simulink model "Sim"  (R2023a)
settings: Solver=FixedStepAuto  StartTime=0.0  StopTime=20  FixedStep=1e-4  RelTol=1e-3
values from neighbouring files (symbols this model uses):
  A1 = 28e-4    (= 0.0028)    [main.m]    (also in main2.m; main3.m; main4.m)
  a1 = 0.071e-4    (= 7.1e-06)    [main.m]    (also in main2.m; main3.m; main4.m)
  A2 = 32e-4    (= 0.0032)    [main.m]    (also in main2.m; main3.m; main4.m)
  a2 = 0.057e-4    (= 5.7e-06)    [main.m]    (also in main2.m; main3.m; main4.m)
  a3 = 0.071e-4    (= 7.1e-06)    [main.m]    (also in main2.m; main3.m; main4.m)
  A3 = 28e-4    (= 0.0028)    [main.m]    (also in main2.m; main3.m; main4.m)
  A4 = 32e-4    (= 0.0032)    [main.m]    (also in main2.m; main3.m; main4.m)
  a4 = 0.057e-4    (= 5.7e-06)    [main.m]    (also in main2.m; main3.m; main4.m)
  Com_V1 = 1.1*V01    (= 3.3)    [main.m]
  Com_V2 = 1.1*V02    (= 3.3)    [main.m]
  delay_Com_V1 = 2.5    [main.m]
  delay_Com_V2 = 1.5    [main.m]
  g = 9.81    [main.m]    (also in main2.m; main3.m; main4.m)
  gamma1 = 0.7    [main.m]    (also in main2.m; main3.m; main4.m)
  gamma2 = 0.6    [main.m]    (also in main2.m; main3.m; main4.m)
  H01 = (gamma1*k1*V01+(1-gamma2)*k2*V02)/(a1*sqrt(2*g))    [main.m]    (also in main2.m; main3.m; main4.m)
  H02 = (gamma2*k2*V02+(1-gamma1)*k1*V01)/(a2*sqrt(2*g))    [main.m]    (also in main2.m; main3.m; main4.m)
  H03 = (1-gamma2)*k2*V02/(a3*sqrt(2*g))    [main.m]    (also in main2.m; main3.m; main4.m)
  H04 = (1-gamma1)*k1*V01/(a4*sqrt(2*g))    [main.m]    (also in main2.m; main3.m; main4.m)
  k1 = 3.33e-6    (= 3.33e-06)    [main.m]    (also in main2.m; main3.m; main4.m)
  k2 = 3.35e-6    (= 3.35e-06)    [main.m]    (also in main2.m; main3.m; main4.m)
  Matrix_dX_U = [gamma1*k1/A1, 0 ... (first row only)    [main.m]    (also in main2.m; main3.m; main4.m)
  Matrix_dX_X = [-1/T1, 0, -A3/(A1*T3), 0 ... (first row only)    [main.m]    (also in main2.m; main3.m; main4.m)
  Matrix_H0 = [H01^2;H02^2;H03^2;H04^2]    [main.m]    (also in main2.m; main3.m; main4.m)
  Matrix_V0 = [V01;V02]    [main.m]    (also in main2.m; main3.m; main4.m)
  V01 = 3    [main.m]    (also in main2.m; main3.m; main4.m)
  V02 = 3    [main.m]    (also in main2.m; main3.m; main4.m)
settings Model: Creator=philippecasteres  LastModifiedBy=philippecasteres

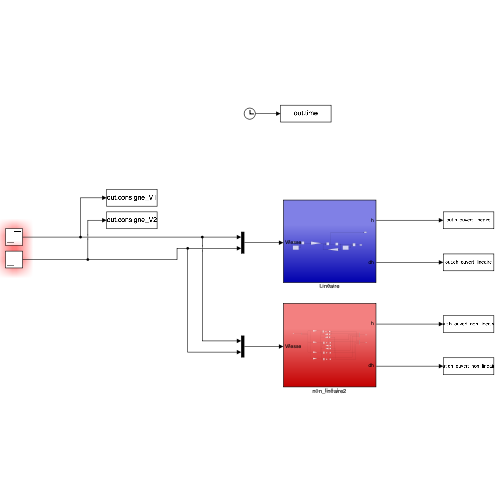
[thumbnail: Simulink's stored preview of the top-level diagram]
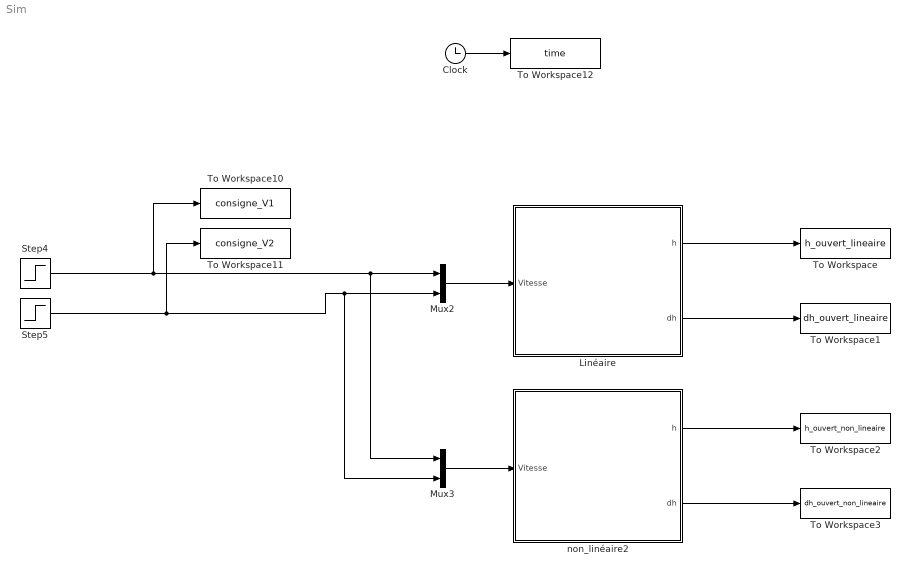
== system Sim ==
  Clock : Clock
  Linéaire : Subsystem
  Mux2 : Mux  Inputs=2
  Mux3 : Mux  Inputs=2
  Step4 : Step  Time=delay_Com_V1  Before=V01  After=Com_V1  SampleTime=0
  Step5 : Step  Time=delay_Com_V2  Before=V02  After=Com_V2  SampleTime=0
  To Workspace : ToWorkspace  VariableName=h_ouvert_lineaire  SaveFormat=Timeseries  SampleTime=-1
  To Workspace1 : ToWorkspace  VariableName=dh_ouvert_lineaire  SaveFormat=Timeseries  SampleTime=-1
  To Workspace10 : ToWorkspace  VariableName=consigne_V1  SaveFormat=Timeseries  SampleTime=-1
  To Workspace11 : ToWorkspace  VariableName=consigne_V2  SaveFormat=Timeseries  SampleTime=-1
  To Workspace12 : ToWorkspace  VariableName=time  SaveFormat=Timeseries  SampleTime=-1
  To Workspace2 : ToWorkspace  VariableName=h_ouvert_non_lineaire  SaveFormat=Timeseries  SampleTime=-1
  To Workspace3 : ToWorkspace  VariableName=dh_ouvert_non_lineaire  SaveFormat=Timeseries  SampleTime=-1
  non_linéaire2 : Subsystem
  wires:
  Step5/1 -> To Workspace11/1, Mux3/2, Mux2/2
  Step4/1 -> To Workspace10/1, Mux3/1, Mux2/1
  Linéaire/1(h) -> To Workspace/1
  Linéaire/2(dh) -> To Workspace1/1
  Mux2/1 -> Linéaire/1(Vitesse)
  non_linéaire2/2(dh) -> To Workspace3/1
  non_linéaire2/1(h) -> To Workspace2/1
  Mux3/1 -> non_linéaire2/1(Vitesse)
  Clock/1 -> To Workspace12/1

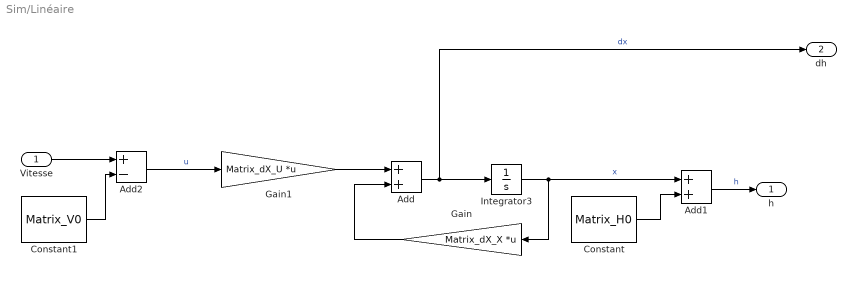
== system Sim/Linéaire ==
  Vitesse : Inport
  Add : Sum
  Add1 : Sum
  Add2 : Sum  Inputs=+-
  Constant : Constant  Value=Matrix_H0
  Constant1 : Constant  Value=Matrix_V0
  Gain : Gain  Gain=Matrix_dX_X  Multiplication=Matrix(K*u)
  Gain1 : Gain  Gain=Matrix_dX_U  Multiplication=Matrix(K*u) (u vector)
  Integrator3 : Integrator
  h : Outport
  dh : Outport  Port=2
  wires:
  Constant/1 -> Add1/2
  Add1/1 -> h/1  "h"
  Add2/1 -> Gain1/1  "u"
  Vitesse/1 -> Add2/1
  Gain/1 -> Add/2
  Constant1/1 -> Add2/2
  Gain1/1 -> Add/1
  Add/1 -> Integrator3/1, dh/1  "dx"
  Integrator3/1 -> Add1/1, Gain/1  "x"

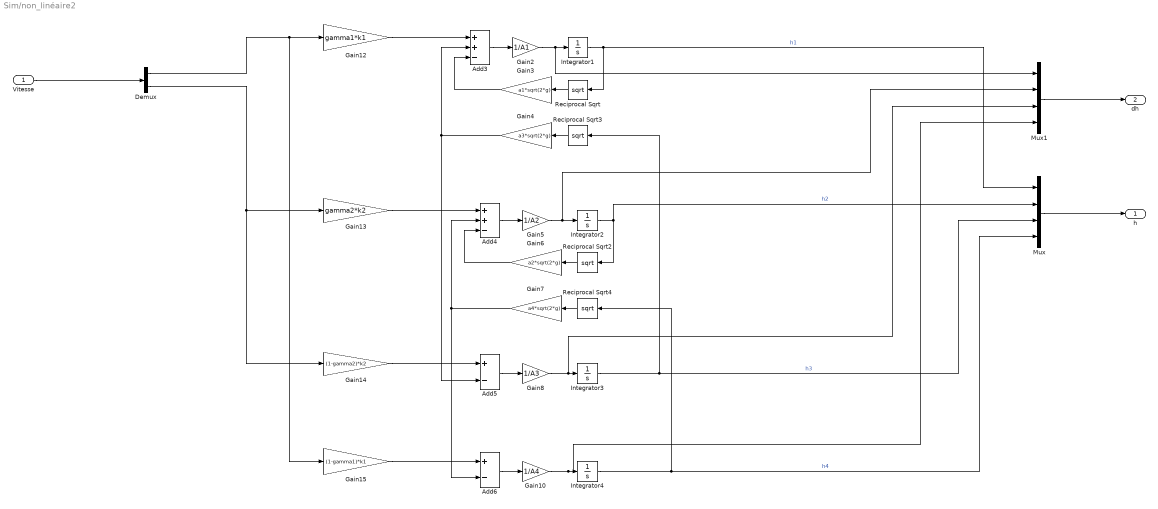
== system Sim/non_linéaire2 ==
  Vitesse : Inport
  Add3 : Sum  Inputs=++-
  Add4 : Sum  Inputs=++-
  Add5 : Sum  Inputs=+-
  Add6 : Sum  Inputs=+-
  Demux : Demux  Outputs=2
  Gain10 : Gain  Gain=1/A4
  Gain12 : Gain  Gain=gamma1*k1
  Gain13 : Gain  Gain=gamma2*k2
  Gain14 : Gain  Gain=(1-gamma2)*k2
  Gain15 : Gain  Gain=(1-gamma1)*k1
  Gain2 : Gain  Gain=1/A1
  Gain3 : Gain  Gain=a1*sqrt(2*g)
  Gain4 : Gain  Gain=a3*sqrt(2*g)
  Gain5 : Gain  Gain=1/A2
  Gain6 : Gain  Gain=a2*sqrt(2*g)
  Gain7 : Gain  Gain=a4*sqrt(2*g)
  Gain8 : Gain  Gain=1/A3
  Integrator1 : Integrator  InitialCondition=H01^2
  Integrator2 : Integrator  InitialCondition=H02^2
  Integrator3 : Integrator  InitialCondition=H03^2
  Integrator4 : Integrator  InitialCondition=H04^2
  Mux : Mux
  Mux1 : Mux
  Reciprocal Sqrt{,2..4} (4 alike) : Sqrt
  h : Outport
  dh : Outport  Port=2
  wires:
  Add3/1 -> Gain2/1
  Gain2/1 -> Mux1/1, Integrator1/1
  Integrator1/1 -> Reciprocal Sqrt/1, Mux/1  "h1"
  Gain3/1 -> Add3/3
  Gain4/1 -> Add5/2, Add3/2
  Reciprocal Sqrt/1 -> Gain3/1
  Gain6/1 -> Add4/3
  Gain5/1 -> Mux1/2, Integrator2/1
  Add4/1 -> Gain5/1
  Integrator2/1 -> Mux/2, Reciprocal Sqrt2/1  "h2"
  Reciprocal Sqrt2/1 -> Gain6/1
  Gain7/1 -> Add6/2, Add4/2
  Add5/1 -> Gain8/1
  Reciprocal Sqrt3/1 -> Gain4/1
  Gain8/1 -> Mux1/3, Integrator3/1
  Integrator3/1 -> Mux/3, Reciprocal Sqrt3/1  "h3"
  Reciprocal Sqrt4/1 -> Gain7/1
  Integrator4/1 -> Mux/4, Reciprocal Sqrt4/1  "h4"
  Gain10/1 -> Mux1/4, Integrator4/1
  Add6/1 -> Gain10/1
  Mux/1 -> h/1
  Mux1/1 -> dh/1
  Gain12/1 -> Add3/1
  Gain13/1 -> Add4/1
  Gain15/1 -> Add6/1
  Gain14/1 -> Add5/1
  Demux/1 -> Gain15/1, Gain12/1
  Demux/2 -> Gain14/1, Gain13/1
  Vitesse/1 -> Demux/1
